simulink model "Angle_from_sensor_models"  (R2020b)
settings: Solver=FixedStepAuto  StartTime=0.0  StopTime=inf  RelTol=1e-3
settings Model: SILPILModeSetting=veronly  ExtModeTrigDuration=2  Creator=Abdou  LastModifiedBy=Abdou
settings OptimizationCC: EnhancedBackFolding=on  PassReuseOutputArgsAs=Individual arguments  ZeroExternalMemoryAtStartup=off  ZeroInternalMemoryAtStartup=off  MaxStackSize=64  OptimizeBlockOrder=speed  DifferentSizesBufferReuse=on  OptimizationCustomize=off  EfficientTunableParamExpr=on
settings DebuggingCC: ParameterTunabilityLossMsg=error
settings HardwareCC: ProdBitPerInt=16  ProdBitPerPointer=16  ProdBitPerSizeT=16  ProdBitPerPtrDiffT=16  ProdLargestAtomicFloat=None  ProdWordSize=8  ProdHWDeviceType=Atmel->AVR
settings SFSimCC: MATLABDynamicMemAlloc=off
settings RTWCC: Description=Embedded Coder  SystemTargetFile=ert.tlc  HardwareBoard=Arduino Uno  TemplateMakefile=ert_default_tmf  Toolchain=Arduino AVR
settings CodeAppCC: ForceParamTrailComments=on  IgnoreCustomStorageClasses=off  OperatorAnnotations=on  SimulinkDataObjDesc=on  SFDataObjDesc=on  InsertBlockDesc=on
settings ERTTargetCC: SupportContinuousTime=on  SupportVariableSizeSignals=on  ExtMode=on  ExtModeStaticAllocSize=250  ExtModeMexArgs='127.0.0.1' 0 17725

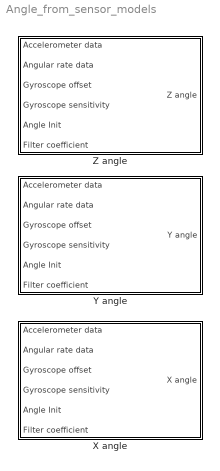
== system Angle_from_sensor_models ==
  X angle : Subsystem
  Y angle : Subsystem
  Z angle : Subsystem

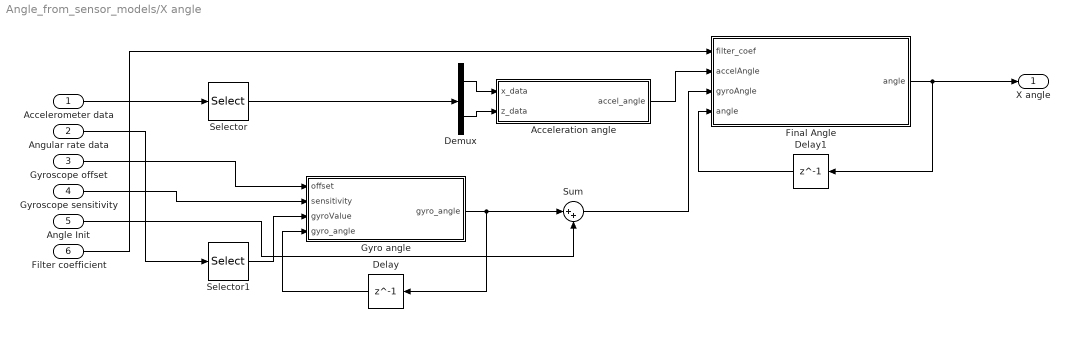
== system Angle_from_sensor_models/X angle ==
  Accelerometer data : Inport
  Angular rate data : Inport  Port=2
  Gyroscope offset : Inport  Port=3
  Gyroscope sensitivity : Inport  Port=4
  Angle Init : Inport  Port=5
  Filter coefficient : Inport  Port=6
  Acceleration angle : MATLAB Function  TreatAsAtomicUnit=on
  Delay : Delay  DelayLength=1  InitialCondition=0
  Delay1 : Delay  DelayLength=1  InitialCondition=0
  Demux : Demux  Outputs=2
  Final Angle : MATLAB Function  TreatAsAtomicUnit=on
  Gyro angle : MATLAB Function  TreatAsAtomicUnit=on
  Selector : Selector  InputPortWidth=3  IndexOptions=Index vector (dialog)  Indices=[2 3]  OutputSizes=1
  Selector1 : Selector  InputPortWidth=3  IndexOptions=Index vector (dialog)  Indices=1  OutputSizes=1
  Sum : Sum  Inputs=|++
  X angle : Outport
  wires:
  Demux/1 -> Acceleration angle/1(x_data)
  Sum/1 -> Final Angle/3(gyroAngle)
  Delay/1 -> Gyro angle/4("gyro_angle ")
  Angle Init/1 -> Sum/2
  Demux/2 -> Acceleration angle/2(z_data)
  Gyro angle/1(gyro_angle) -> Sum/1, Delay/1
  Selector1/1 -> Gyro angle/3(gyroValue)
  Final Angle/1(angle) -> X angle/1, Delay1/1
  Filter coefficient/1 -> Final Angle/1(filter_coef)
  Selector/1 -> Demux/1
  Acceleration angle/1(accel_angle) -> Final Angle/2(accelAngle)
  Delay1/1 -> Final Angle/4("angle ")
  Gyroscope sensitivity/1 -> Gyro angle/2(sensitivity)
  Accelerometer data/1 -> Selector/1
  Angular rate data/1 -> Selector1/1
  Gyroscope offset/1 -> Gyro angle/1(offset)

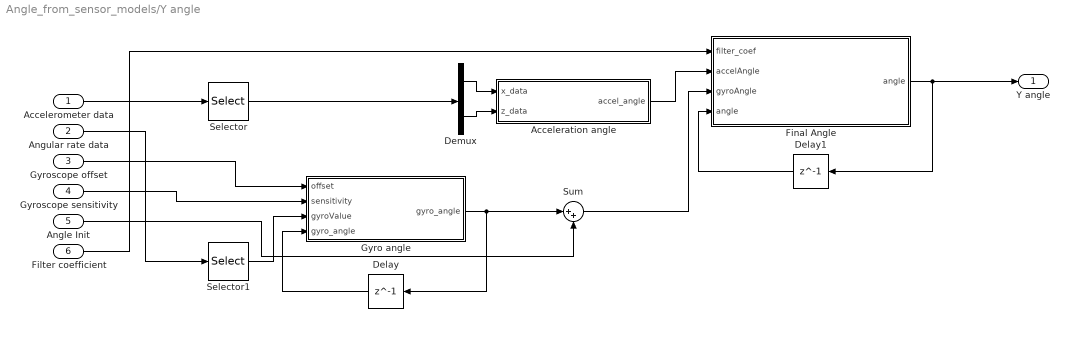
== system Angle_from_sensor_models/Y angle ==
  Accelerometer data : Inport
  Angular rate data : Inport  Port=2
  Gyroscope offset : Inport  Port=3
  Gyroscope sensitivity : Inport  Port=4
  Angle Init : Inport  Port=5
  Filter coefficient : Inport  Port=6
  Acceleration angle : MATLAB Function  TreatAsAtomicUnit=on
  Delay : Delay  DelayLength=1  InitialCondition=0
  Delay1 : Delay  DelayLength=1  InitialCondition=0
  Demux : Demux  Outputs=2
  Final Angle : MATLAB Function  TreatAsAtomicUnit=on
  Gyro angle : MATLAB Function  TreatAsAtomicUnit=on
  Selector : Selector  InputPortWidth=3  IndexOptions=Index vector (dialog)  Indices=[1 3]  OutputSizes=1
  Selector1 : Selector  InputPortWidth=3  IndexOptions=Index vector (dialog)  Indices=2  OutputSizes=1
  Sum : Sum  Inputs=|++
  Y angle : Outport
  wires:
  Demux/1 -> Acceleration angle/1(x_data)
  Sum/1 -> Final Angle/3(gyroAngle)
  Delay/1 -> Gyro angle/4("gyro_angle ")
  Angle Init/1 -> Sum/2
  Demux/2 -> Acceleration angle/2(z_data)
  Gyro angle/1(gyro_angle) -> Sum/1, Delay/1
  Selector1/1 -> Gyro angle/3(gyroValue)
  Final Angle/1(angle) -> Y angle/1, Delay1/1
  Filter coefficient/1 -> Final Angle/1(filter_coef)
  Selector/1 -> Demux/1
  Acceleration angle/1(accel_angle) -> Final Angle/2(accelAngle)
  Delay1/1 -> Final Angle/4("angle ")
  Gyroscope sensitivity/1 -> Gyro angle/2(sensitivity)
  Accelerometer data/1 -> Selector/1
  Angular rate data/1 -> Selector1/1
  Gyroscope offset/1 -> Gyro angle/1(offset)

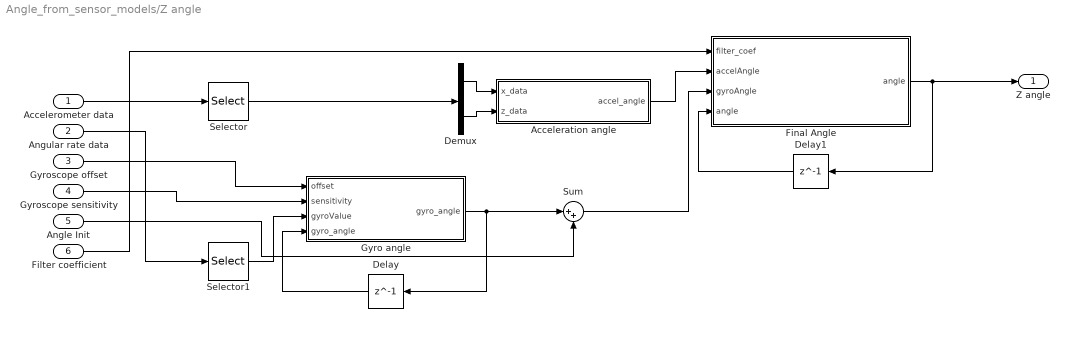
== system Angle_from_sensor_models/Z angle ==
  Accelerometer data : Inport
  Angular rate data : Inport  Port=2
  Gyroscope offset : Inport  Port=3
  Gyroscope sensitivity : Inport  Port=4
  Angle Init : Inport  Port=5
  Filter coefficient : Inport  Port=6
  Acceleration angle : MATLAB Function  TreatAsAtomicUnit=on
  Delay : Delay  DelayLength=1  InitialCondition=0
  Delay1 : Delay  DelayLength=1  InitialCondition=0
  Demux : Demux  Outputs=2
  Final Angle : MATLAB Function  TreatAsAtomicUnit=on
  Gyro angle : MATLAB Function  TreatAsAtomicUnit=on
  Selector : Selector  InputPortWidth=3  IndexOptions=Index vector (dialog)  Indices=[1 2]  OutputSizes=1
  Selector1 : Selector  InputPortWidth=3  IndexOptions=Index vector (dialog)  Indices=3  OutputSizes=1
  Sum : Sum  Inputs=|++
  Z angle : Outport
  wires:
  Demux/1 -> Acceleration angle/1(x_data)
  Sum/1 -> Final Angle/3(gyroAngle)
  Delay/1 -> Gyro angle/4("gyro_angle ")
  Angle Init/1 -> Sum/2
  Demux/2 -> Acceleration angle/2(z_data)
  Gyro angle/1(gyro_angle) -> Sum/1, Delay/1
  Selector1/1 -> Gyro angle/3(gyroValue)
  Final Angle/1(angle) -> Z angle/1, Delay1/1
  Filter coefficient/1 -> Final Angle/1(filter_coef)
  Selector/1 -> Demux/1
  Acceleration angle/1(accel_angle) -> Final Angle/2(accelAngle)
  Delay1/1 -> Final Angle/4("angle ")
  Gyroscope sensitivity/1 -> Gyro angle/2(sensitivity)
  Accelerometer data/1 -> Selector/1
  Angular rate data/1 -> Selector1/1
  Gyroscope offset/1 -> Gyro angle/1(offset)

== matlab function Angle_from_sensor_models/Z angle/Final Angle ==
  data: filter_coef input; accelAngle input; gyroAngle input; angle output; angle input
function angle = Complimentary_filter(filter_coef,accelAngle,gyroAngle,angle)
    angle = filter_coef * (angle + gyroAngle / 100 ) + (1 - filter_coef) * accelAngle;

== matlab function Angle_from_sensor_models/Z angle/Gyro angle ==
  data: offset input; sensitivity input; gyroValue input; gyro_angle output; gyro_angle input
function gyro_angle = Gyro_angle(offset,sensitivity,gyroValue,gyro_angle)
    gyroRate = (gyroValue - offset) * sensitivity;
    gyro_angle = gyro_angle - gyroRate / 100.0;

== matlab function Angle_from_sensor_models/Z angle/Acceleration angle ==
  data: x_data input; z_data input; accel_angle output
function accel_angle = Accel_angle(x_data,z_data)
    accel_angle = atan2(x_data,z_data) * 180/pi ;

== matlab function Angle_from_sensor_models/Y angle/Acceleration angle ==
  data: x_data input; z_data input; accel_angle output
function accel_angle = Accel_angle(x_data,z_data)
    accel_angle = atan2(x_data,z_data) * 180/pi ;

== matlab function Angle_from_sensor_models/Y angle/Final Angle ==
  data: filter_coef input; accelAngle input; gyroAngle input; angle output; angle input
function angle = Complimentary_filter(filter_coef,accelAngle,gyroAngle,angle)
    angle = filter_coef * (angle + gyroAngle / 100 ) + (1 - filter_coef) * accelAngle;

== matlab function Angle_from_sensor_models/Y angle/Gyro angle ==
  data: offset input; sensitivity input; gyroValue input; gyro_angle output; gyro_angle input
function gyro_angle = Gyro_angle(offset,sensitivity,gyroValue,gyro_angle)
    gyroRate = (gyroValue - offset) * sensitivity;
    gyro_angle = gyro_angle - gyroRate / 100.0;

== matlab function Angle_from_sensor_models/X angle/Acceleration angle ==
  data: x_data input; z_data input; accel_angle output
function accel_angle = Accel_angle(x_data,z_data)
    accel_angle = atan2(x_data,z_data) * 180/pi ;

== matlab function Angle_from_sensor_models/X angle/Final Angle ==
  data: filter_coef input; accelAngle input; gyroAngle input; angle output; angle input
function angle = Complimentary_filter(filter_coef,accelAngle,gyroAngle,angle)
    angle = filter_coef * (angle + gyroAngle / 100 ) + (1 - filter_coef) * accelAngle;

== matlab function Angle_from_sensor_models/X angle/Gyro angle ==
  data: offset input; sensitivity input; gyroValue input; gyro_angle output; gyro_angle input
function gyro_angle = Gyro_angle(offset,sensitivity,gyroValue,gyro_angle)
    gyroRate = (gyroValue - offset) * sensitivity;
    gyro_angle = gyro_angle - gyroRate / 100.0;
